simulink library "SatelliteLibrary"  (R2017b)
settings: Solver=VariableStepAuto  StartTime=0.0  StopTime=10.0  RelTol=1e-3
libraries: SatelliteLibrary x1
settings Model: Creator=Huib  LastModifiedBy=Huib

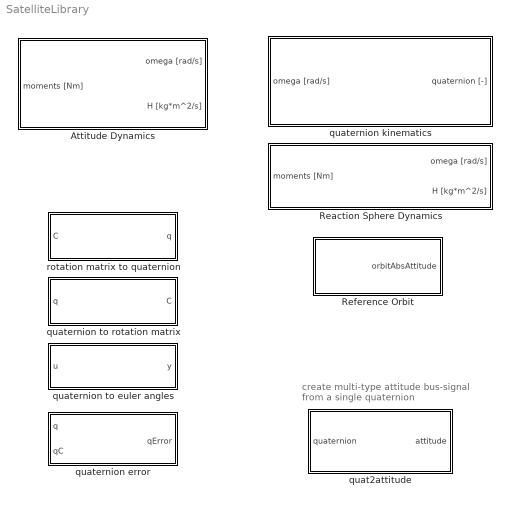
== system SatelliteLibrary ==
  note: create multi-type attitude bus-signal
      | from a single quaternion
  Attitude Dynamics : Subsystem  mask{J11=1.5, J22=1, J33=0.5, omega0=[0.0 0.5 0.01]}
      mask prompts: J11 "J_11"; J22 "J_22"; J33 "J_33"; omega0 "Initial rotational velocity [rad/s]"
      mask DialogControl DescTextVar Prompt: 3-D attitude dynamics along principle axes of body
      mask DialogControl Control2 Prompt: Principle moments of inertia [kg*m^2]
  Reaction Sphere Dynamics : Subsystem  mask{J=0.005567928416632, omega0=[0 0 0]}
      mask prompts: J "Moment of Inertia [kg*m^2]"; omega0 "Initial angular velocity [rad/s]"
      mask DialogControl DescTextVar Prompt: Reaction sphere dynamics.
  Reference Orbit : Subsystem  mask{orbitAltitude=700, gravParam=398600.4418, planetRadius=6371}
      mask prompts: orbitAltitude "Orbital altitude [km]"; gravParam "Gravitational parameter [km^3/s^2]"; planetRadius "Planet radius [km]"
      mask init:
      | orbitFrequency = sqrt(gravParam / (orbitAltitude + planetRadius)^3)
      mask DialogControl DescTextVar Prompt: Outputs rotation amtrix and quaternion describing orientation of frame in a circular orbit w.r.t. inertial space.
  quat2attitude : Subsystem
  quaternion error : MATLAB Function  TreatAsAtomicUnit=on
  quaternion kinematics : Subsystem  mask{q_0=[0 0 0 1]}
      mask prompts: q_0 "Initial quaternion rotation"
      mask DialogControl DescTextVar Prompt: Quaternion attitude kinematic differential equation
  quaternion to euler angles : MATLAB Function  TreatAsAtomicUnit=on
  quaternion to rotation matrix : MATLAB Function  TreatAsAtomicUnit=on
  rotation matrix to quaternion : MATLAB Function  TreatAsAtomicUnit=on

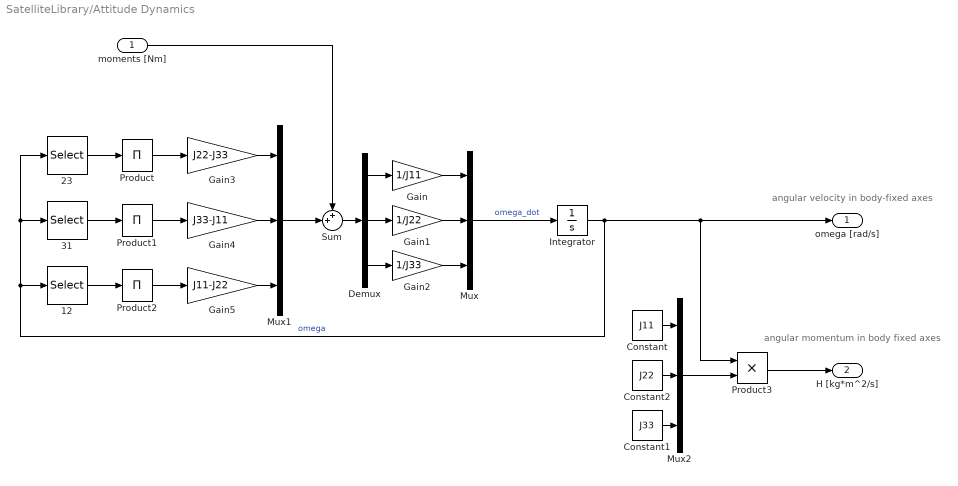
== system SatelliteLibrary/Attitude Dynamics ==
  note: angular momentum in body fixed axes
  note: angular velocity in body-fixed axes
  moments [Nm] : Inport  PortDimensions=3
  12 : Selector  InputPortWidth=3  IndexOptions=Index vector (dialog)  Indices=[1 2]  OutputSizes=1
  23 : Selector  InputPortWidth=3  IndexOptions=Index vector (dialog)  Indices=[2 3]  OutputSizes=1
  31 : Selector  InputPortWidth=3  IndexOptions=Index vector (dialog)  Indices=[3 1]  OutputSizes=1
  Constant : Constant  Value=J11
  Constant1 : Constant  Value=J33
  Constant2 : Constant  Value=J22
  Demux : Demux  Outputs=3
  Gain : Gain  Gain=1/J11
  Gain1 : Gain  Gain=1/J22
  Gain2 : Gain  Gain=1/J33
  Gain3 : Gain  Gain=J22-J33
  Gain4 : Gain  Gain=J33-J11
  Gain5 : Gain  Gain=J11-J22
  Integrator : Integrator  InitialCondition=omega0
  Mux : Mux  Inputs=3
  Mux1 : Mux  Inputs=3
  Mux2 : Mux  Inputs=3
  Product : Product  Inputs=1
  Product1 : Product  Inputs=1
  Product2 : Product  Inputs=1
  Product3 : Product
  Sum : Sum  Inputs=++|
  omega [rad/s] : Outport
  H [kg*m^2/s] : Outport  Port=2
  wires:
  Integrator/1 -> Product3/1, omega [rad/s]/1, 23/1, 31/1, 12/1  "omega"
  Product/1 -> Gain3/1
  Gain3/1 -> Mux1/1
  31/1 -> Product1/1
  12/1 -> Product2/1
  23/1 -> Product/1
  Product2/1 -> Gain5/1
  Gain5/1 -> Mux1/3
  Product1/1 -> Gain4/1
  Gain4/1 -> Mux1/2
  moments [Nm]/1 -> Sum/1
  Mux1/1 -> Sum/2
  Sum/1 -> Demux/1
  Demux/1 -> Gain/1
  Demux/3 -> Gain2/1
  Demux/2 -> Gain1/1
  Mux/1 -> Integrator/1  "omega_dot"
  Gain2/1 -> Mux/3
  Gain/1 -> Mux/1
  Gain1/1 -> Mux/2
  Constant/1 -> Mux2/1
  Constant2/1 -> Mux2/2
  Constant1/1 -> Mux2/3
  Mux2/1 -> Product3/2
  Product3/1 -> H [kg*m^2/s]/1

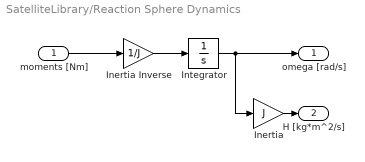
== system SatelliteLibrary/Reaction Sphere Dynamics ==
  moments [Nm] : Inport
  Inertia : Gain  Gain=J
  Inertia Inverse : Gain  Gain=1/J
  Integrator : Integrator  InitialCondition=omega0
  omega [rad/s] : Outport
  H [kg*m^2/s] : Outport  Port=2
  wires:
  moments [Nm]/1 -> Inertia Inverse/1
  Inertia Inverse/1 -> Integrator/1
  Integrator/1 -> Inertia/1, omega [rad/s]/1
  Inertia/1 -> H [kg*m^2/s]/1

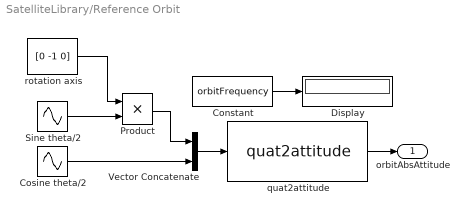
== system SatelliteLibrary/Reference Orbit ==
  Constant : Constant  Value=orbitFrequency
  Cosine theta/2 : Sin  Frequency=orbitFrequency/2  Phase=pi/2  SampleTime=0
  Display : Display
  Product : Product
  Sine theta/2 : Sin  Frequency=orbitFrequency/2  SampleTime=0
  Vector Concatenate : Concatenate
  quat2attitude : SatelliteLibrary/quat2attitude
  rotation axis : Constant  Value=[0 -1 0]
  orbitAbsAttitude : Outport
  wires:
  Product/1 -> Vector Concatenate/1
  rotation axis/1 -> Product/1
  Sine theta/2/1 -> Product/2
  Cosine theta/2/1 -> Vector Concatenate/2
  Vector Concatenate/1 -> quat2attitude/1
  Constant/1 -> Display/1
  quat2attitude/1 -> orbitAbsAttitude/1

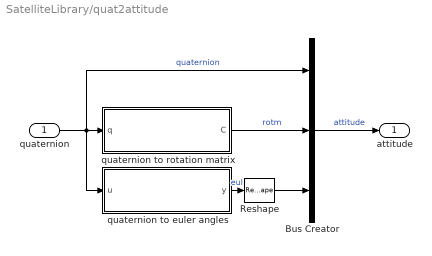
== system SatelliteLibrary/quat2attitude ==
  quaternion : Inport
  Bus Creator : BusCreator  Inputs=3
  Reshape : Reshape
  quaternion to euler angles : MATLAB Function  TreatAsAtomicUnit=on
  quaternion to rotation matrix : MATLAB Function  TreatAsAtomicUnit=on
  attitude : Outport
  wires:
  quaternion to rotation matrix/1(C) -> Bus Creator/2  "rotm"
  Bus Creator/1 -> attitude/1  "attitude"
  quaternion to euler angles/1(y) -> Reshape/1  "eul"
  quaternion/1 -> quaternion to euler angles/1(u), quaternion to rotation matrix/1(q), Bus Creator/1  "quaternion"
  Reshape/1 -> Bus Creator/3

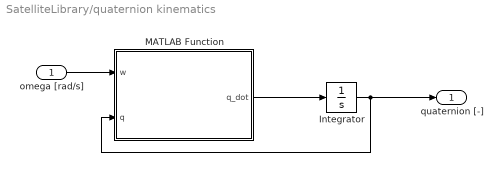
== system SatelliteLibrary/quaternion kinematics ==
  omega [rad/s] : Inport
  Integrator : Integrator  InitialCondition=q_0
  MATLAB Function : MATLAB Function  TreatAsAtomicUnit=on
  quaternion [-] : Outport
  wires:
  MATLAB Function/1(q_dot) -> Integrator/1
  Integrator/1 -> quaternion [-]/1, MATLAB Function/2(q)
  omega [rad/s]/1 -> MATLAB Function/1(w)

== matlab function SatelliteLibrary/quaternion to rotation matrix ==
  data: q input; C output
function C = quat2rotm(q)
% Convert quaternion q to a rotation matrix C (in vector form)
% q is a standard quaternion with the vector part at the start
% C is a 9x1 vector with elements[Column1; Column2; Column3]

x = q(1);
y = q(2);
z = q(3);
s = q(4);

C = [1-2*(y^2 + z^2),   2*(y*x - z*s),   2*(z*x + y*s);...
       2*(x*y + z*s), 1-2*(x^2 + z^2),   2*(z*y - x*s);...
       2*(x*z - y*s),   2*(y*z + x*s), 1-2*(x^2 + y^2)];
end

== matlab function SatelliteLibrary/rotation matrix to quaternion ==
  data: C input; q output
function q = rotm2quat(C)
% Convert rotation matrix C (in vector form) to a quaternion q
% C is a 3x3 rotation matrix
% q is a standard quaternion with the vector part at the start

% Method according to 
%       I.Y. Bar-Itzhack, "New method for extracting the quaternion from a 
%       rotation matrix," Journal of Guidance, Control, and Dynamics, 
%       vol. 23, no. 6, pp. 1085-1087, 2000
% Using basically the same code as rotm2quat from robotics toolbox

% Calculate all elements of symmetric K matrix
K11 = C(1,1) - C(2,2) - C(3,3);
K12 = C(1,2) + C(2,1);
K13 = C(1,3) + C(3,1);
K14 = C(3,2) - C(2,3);

K22 = C(2,2) - C(1,1) - C(3,3);
K23 = C(2,3) + C(3,2);
K24 = C(1,3) - C(3,1);

K33 = C(3,3) - C(1,1) - C(2,2);
K34 = C(2,1) - C(1,2);

K44 = C(1,1) + C(2,2) + C(3,3);

% Construct K matrix according to paper
K = [K11,    K12,    K13,    K14;
     K12,    K22,    K23,    K24;
     K13,    K23,    K33,    K34;
     K14,    K24,    K34,    K44];

K = K ./ 3;
[eigVec, eigVal] = eig(K, 'vector');
[~, maxIndex] = max(real(eigVal));
q = real(eigVec(:,maxIndex));
if q(4)<0
   q = -q; 
end
end

== matlab function SatelliteLibrary/quaternion kinematics/MATLAB Function ==
  data: w input; q_dot output; q input
function q_dot = omega2qdot(w, q)
% Kinematics for converting body-fixed rotation rates omega to quaternion
% derivative q_dot
q_dot = [...
    w(1)*q(4) - w(2)*q(3) + w(3)*q(2);...
    w(1)*q(3) + w(2)*q(4) - w(3)*q(1);...
    w(3)*q(4) + w(2)*q(1) - w(1)*q(2);...
   -q(1)*w(1) - q(2)*w(2) - q(3)*w(3)];
q_dot = q_dot ./ 2;
end

== matlab function SatelliteLibrary/quat2attitude/quaternion to euler angles ==
  data: u input; y output
function y = quat2eul(u)
q = [u(4); u(1:3)];
y = quat2eul(q', 'ZYX');
end

== matlab function SatelliteLibrary/quaternion error ==
  data: q input; qError output; qC input
function qError = quatError(...
    q, ... current quaternion orientation
    qC ... desired quaternion orientation
    )
% Calculate the error quaternion
% q_... are standard quaternions with the vector part at the start

qCmatrix = [ qC(4)  qC(3) -qC(2) -qC(1);...
            -qC(3)  qC(4)  qC(1) -qC(2);...
             qC(2) -qC(1)  qC(4) -qC(3);...
             qC(1)  qC(2)  qC(3)  qC(4)];
qError = qCmatrix * q;
end

== matlab function SatelliteLibrary/quaternion to euler angles ==
  data: u input; y output
function y = quat2eul(u)
q = [u(4); u(1:3)];
y = quat2eul(q', 'ZYX');
end

== matlab function SatelliteLibrary/quat2attitude/quaternion to rotation matrix ==
  data: q input; C output
function C = quat2rotm(q)
% Convert quaternion q to a rotation matrix C (in vector form)
% q is a standard quaternion with the vector part at the start
% C is a 9x1 vector with elements[Column1; Column2; Column3]

x = q(1);
y = q(2);
z = q(3);
s = q(4);

C = [1-2*(y^2 + z^2),   2*(y*x - z*s),   2*(z*x + y*s);...
       2*(x*y + z*s), 1-2*(x^2 + z^2),   2*(z*y - x*s);...
       2*(x*z - y*s),   2*(y*z + x*s), 1-2*(x^2 + y^2)];
end
